simulink model "PowetrainModel"  (R2020b)
settings: Solver=VariableStepAuto  StartTime=0.0  StopTime=10.0  RelTol=1e-3
undefined symbols (not defined in the file or in its folder): sigbuilder_block
settings Model: Creator=joems  LastModifiedBy=joems

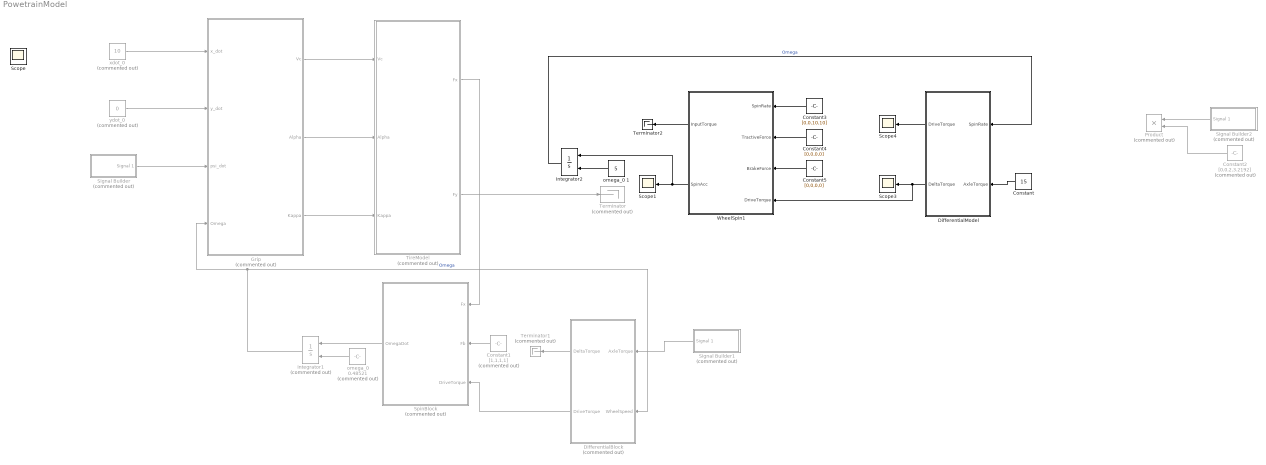
== system PowetrainModel ==
  Constant : Constant  Value=15
  Constant1 : Constant  Commented=on  Value=[1,1,1,1]
  Constant2 : Constant  Commented=on  Value=[0,0,2,3.2192]
  Constant3 : Constant  Value=[0,0,10,10]
  Constant4 : Constant  Value=[0,0,0,0]
  Constant5 : Constant  Value=[0,0,0,0]
  DifferentialBlock : MATLAB Function  Commented=on  TreatAsAtomicUnit=on
  DifferentialModel : MATLAB Function  TreatAsAtomicUnit=on
  Grip : MATLAB Function  Commented=on  TreatAsAtomicUnit=on
  Integrator1 : Integrator  Commented=on  InitialConditionSource=external
  Integrator2 : Integrator  InitialConditionSource=external
  Product : Product  Commented=on
  Scope{,1,3..4} (4 alike) : Scope
  Signal Builder : Subsystem  Tag=STV Subsys  Commented=on  LoadFcn=sigbuilder_block('load');  StartFcn=sigbuilder_block('start');  StopFcn=sigbuilder_block('stop');  ClipboardFcn=sigbuilder_block('clipboard');  mask(Sigbuilder block){tuvar=[0:10]}
      mask help: Simulink:masks:SigbuilderBlock_MD
      mask init:
      | if ~strcmp(get_param(bdroot(gcbh),'SimulationStatus'),'stopped') tuvar = sigbuilder_block('maskInit'); end
      settings: CopyFcn=sigbuilder_block('copy');  DeleteFcn=sigbuilder_block('delete');  ModelCloseFcn=sigbuilder_block('modelClose');  PreSaveFcn=sigbuilder_block('preSave');  PauseFcn=sigbuilder_block('pause');  ContinueFcn=sigbuilder_block('continue');  NameChangeFcn=sigbuilder_block('namechange');  OpenFcn=sigbuilder_block('open',[281.4 118.8 550.8 400.2 ]);  CloseFcn=sigbuilder_block('close');
      mask Display: plot(0, 0, 100, 100,[2, 2, 32, 32, 2], [68, 8, 8, 68, 68],[32, 2], [38, 38], [32, 19, 2],[53, 60, 44], [32, 17, 17, 2],[16, 16, 31, 31]);txt = getActiveGroup(gcbh);text(2, 100, txt,'verticalAlignment', 'top');
  Signal Builder1 : Subsystem  Tag=STV Subsys  Commented=on  LoadFcn=sigbuilder_block('load');  StartFcn=sigbuilder_block('start');  StopFcn=sigbuilder_block('stop');  ClipboardFcn=sigbuilder_block('clipboard');  mask(Sigbuilder block){tuvar=[0:10]}
      mask help: Simulink:masks:SigbuilderBlock_MD
      mask init:
      | if ~strcmp(get_param(bdroot(gcbh),'SimulationStatus'),'stopped') tuvar = sigbuilder_block('maskInit'); end
      settings: CopyFcn=sigbuilder_block('copy');  DeleteFcn=sigbuilder_block('delete');  ModelCloseFcn=sigbuilder_block('modelClose');  PreSaveFcn=sigbuilder_block('preSave');  PauseFcn=sigbuilder_block('pause');  ContinueFcn=sigbuilder_block('continue');  NameChangeFcn=sigbuilder_block('namechange');  OpenFcn=sigbuilder_block('open',[281.4 118.8 550.8 400.2 ]);  CloseFcn=sigbuilder_block('close');
      mask Display: plot(0, 0, 100, 100,[2, 2, 32, 32, 2], [68, 8, 8, 68, 68],[32, 2], [38, 38], [32, 19, 2],[53, 60, 44], [32, 17, 17, 2],[16, 16, 31, 31]);txt = getActiveGroup(gcbh);text(2, 100, txt,'verticalAlignment', 'top');
  Signal Builder2 : Subsystem  Tag=STV Subsys  Commented=on  LoadFcn=sigbuilder_block('load');  StartFcn=sigbuilder_block('start');  StopFcn=sigbuilder_block('stop');  ClipboardFcn=sigbuilder_block('clipboard');  mask(Sigbuilder block){tuvar=[0:10]}
      mask help: Simulink:masks:SigbuilderBlock_MD
      mask init:
      | if ~strcmp(get_param(bdroot(gcbh),'SimulationStatus'),'stopped') tuvar = sigbuilder_block('maskInit'); end
      settings: CopyFcn=sigbuilder_block('copy');  DeleteFcn=sigbuilder_block('delete');  ModelCloseFcn=sigbuilder_block('modelClose');  PreSaveFcn=sigbuilder_block('preSave');  PauseFcn=sigbuilder_block('pause');  ContinueFcn=sigbuilder_block('continue');  NameChangeFcn=sigbuilder_block('namechange');  OpenFcn=sigbuilder_block('open',[281.4 118.8 550.8 400.2 ]);  CloseFcn=sigbuilder_block('close');
      mask Display: plot(0, 0, 100, 100,[2, 2, 32, 32, 2], [68, 8, 8, 68, 68],[32, 2], [38, 38], [32, 19, 2],[53, 60, 44], [32, 17, 17, 2],[16, 16, 31, 31]);txt = getActiveGroup(gcbh);text(2, 100, txt,'verticalAlignment', 'top');
  SpinBlock : MATLAB Function  Commented=on  TreatAsAtomicUnit=on
  Terminator : Terminator  Commented=on
  Terminator1 : Terminator  Commented=on
  Terminator2 : Terminator
  TireModel : MATLAB Function  Commented=on  TreatAsAtomicUnit=on
  WheelSpin1 : MATLAB Function  TreatAsAtomicUnit=on
  "omega_0 " : Constant  Commented=on  Value=0.48521
  omega_0 1 : Constant  Value=5
  xdot_0 : Constant  Commented=on  Value=10
  ydot_0 : Constant  Commented=on  Value=0
  wires:
  Signal Builder/1(Signal 1) -> Grip/3(psi_dot)
  ydot_0/1 -> Grip/2(y_dot)
  xdot_0/1 -> Grip/1(x_dot)
  Grip/1(Vc) -> TireModel/1(Vc)
  Grip/2(Alpha) -> TireModel/2(Alpha)
  Grip/3(Kappa) -> TireModel/3(Kappa)
  TireModel/1(Fx) -> SpinBlock/1(Fx)
  SpinBlock/1(OmegaDot) -> Integrator1/1
  "omega_0 "/1 -> Integrator1/2
  Integrator1/1 -> DifferentialBlock/2(WheelSpeed), Grip/4(Omega)  "Omega"
  TireModel/2(Fy) -> Terminator/1
  Constant1/1 -> SpinBlock/2(Fb)
  Signal Builder1/1(Signal 1) -> DifferentialBlock/1(AxleTorque)
  DifferentialBlock/2(DriveTorque) -> SpinBlock/3(DriveTorque)
  DifferentialBlock/1(DeltaTorque) -> Terminator1/1
  DifferentialModel/1(DriveTorque) -> Scope4/1
  Signal Builder2/1(Signal 1) -> Product/1
  Constant2/1 -> Product/2
  Constant/1 -> DifferentialModel/2(AxleTorque)
  Constant3/1 -> WheelSpin1/1(SpinRate)
  Constant4/1 -> WheelSpin1/2(TractiveForce)
  DifferentialModel/2(DeltaTorque) -> WheelSpin1/4(DriveTorque), Scope3/1
  Constant5/1 -> WheelSpin1/3(BrakeForce)
  WheelSpin1/1(InputTorque) -> Terminator2/1
  omega_0 1/1 -> Integrator2/2
  WheelSpin1/2(SpinAcc) -> Integrator2/1, Scope1/1
  Integrator2/1 -> DifferentialModel/1(SpinRate)  "Omega"

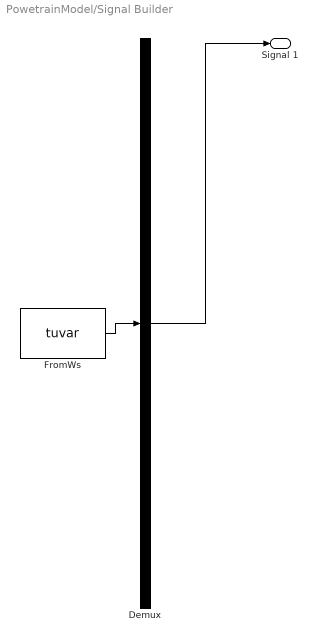
== system PowetrainModel/Signal Builder ==
  Demux : Demux  Tag=STV Demux  Outputs=1
      settings: DisplayOption=none
  FromWs : FromWorkspace  Tag=STV FromWs  VariableName=tuvar
      SigBuilderData=|
      | common.afterFinalStr = 'Extrapolate'
      | common.sampleTime = 0
      | dataSet.timeRange = [0 10]
      | dataSet.name = 'Group 1'
      | sbobj.Groups.Name = 'Group 1'
      | sbobj.Groups.Signals.Name = 'Signal 1'
      | sbobj.Groups.Signals.XData = [0 4 4.3 6 10]
      | sbobj.Groups.Signals.YData = [0 -0.005 1 1 1]
  Signal 1 : Outport  Tag=STV Outport
  wires:
  Demux/1 -> Signal 1/1
  FromWs/1 -> Demux/1

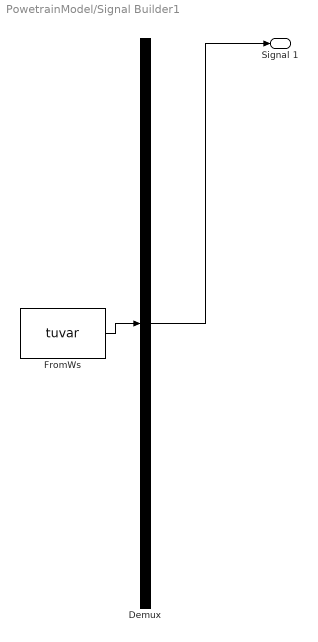
== system PowetrainModel/Signal Builder1 ==
  Demux : Demux  Tag=STV Demux  Outputs=1
      settings: DisplayOption=none
  FromWs : FromWorkspace  Tag=STV FromWs  VariableName=tuvar
      SigBuilderData=|
      | common.afterFinalStr = 'Extrapolate'
      | common.sampleTime = 0
      | dataSet.timeRange = [0 10]
      | dataSet.name = 'Group 1'
      | sbobj.Groups.Name = 'Group 1'
      | sbobj.Groups.Signals.Name = 'Signal 1'
      | sbobj.Groups.Signals.XData = [0 4 4.3 6 10]
      | sbobj.Groups.Signals.YData = [0 -0.005 1 1 1]
  Signal 1 : Outport  Tag=STV Outport
  wires:
  Demux/1 -> Signal 1/1
  FromWs/1 -> Demux/1

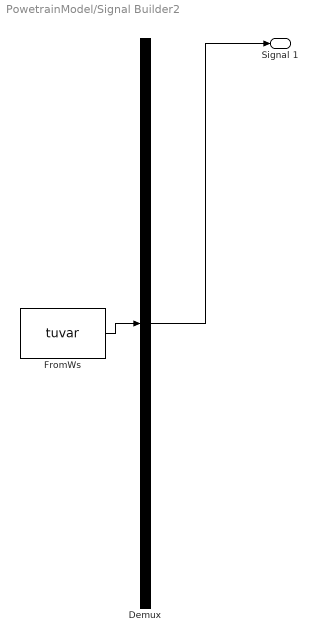
== system PowetrainModel/Signal Builder2 ==
  Demux : Demux  Tag=STV Demux  Outputs=1
      settings: DisplayOption=none
  FromWs : FromWorkspace  Tag=STV FromWs  VariableName=tuvar
      SigBuilderData=|
      | common.afterFinalStr = 'Extrapolate'
      | common.sampleTime = 0
      | dataSet.timeRange = [0 10]
      | dataSet.name = 'Group 1'
      | sbobj.Groups.Name = 'Group 1'
      | sbobj.Groups.Signals.Name = 'Signal 1'
      | sbobj.Groups.Signals.XData = [0 4 4 4.3 6 10]
      | sbobj.Groups.Signals.YData = [0 0 -0.005 1 1 1]
  Signal 1 : Outport  Tag=STV Outport
  wires:
  Demux/1 -> Signal 1/1
  FromWs/1 -> Demux/1

== matlab function PowetrainModel/TireModel ==
  data: Vc input; Alpha input; Fx output; Kappa input; Fy output
function [Fx, Fy] = TireModel(Vc, Alpha, Kappa)


Kxk = 1000;
Kya = 1000;

Fx = Kxk .* Kappa; 

Fy = Kya .* Alpha;

Vc = Vc .*1; 





 %[Fx3, Fy3,~, ~, ~] = Tire.ContactPatchLoads(Alpha, Kappa, 267/4, 12, 2, Vc, 3, Fidelity); %Check if the input values are good 

 %[Fx4, Fy4,~, ~, ~] = Tire.ContactPatchLoads(Alpha, Kappa, 267/4, 12, 2, Vc, 4, Fidelity);
 
% Fx = [Fx3, Fx4];
% Fy = [Fy3, Fy4];
end

== matlab function PowetrainModel/Grip ==
  data: x_dot input; Vc output; y_dot input; psi_dot input; Alpha output; Kappa output; Omega input; Parameter parameter
function [Vc, Alpha, Kappa]= Grip(x_dot,...
    y_dot, psi_dot, Omega, Parameter)

%% Variable Names
%x_dot0 - Intiial logetudinal velocity 
%x_dot - Logetidunal velocity
%y_dot0 - Initial lateral velocity
%y_dot Lateral velocity
%psi_dot - Yaw rate, 
%tw - Track width 
%L - Wheel Base 
%Vc3 & Vc4 - Center velocity of rear tires
%Vc3/4_x/y - Center Velocity components 


%% Center Velocity

Vc = zeros(4,2);
    % Logintidinal Center Velocity 
Vc(3,1) = x_dot - psi_dot.*(Parameter.TrackWidth/2); 

Vc(4,1) = x_dot + psi_dot.*(Parameter.TrackWidth/2);

    % Lateral Center Velocity

Vc(3,2) = y_dot - psi_dot.*Parameter.b;  

Vc(4,2) = y_dot - psi_dot.*Parameter.b;


%% Slip Angle

Alpha = zeros(1,4);

Alpha(3) = - atan2d( (y_dot - Parameter.b.*psi_dot)./ (x_dot + ...
    ( (Parameter.TrackWidth/2).*psi_dot) ), x_dot);                                            
Alpha(4) = - atan2d( (y_dot - Parameter.b.*psi_dot) ./ (x_dot - ...
    ( (Parameter.TrackWidth/2).*psi_dot) ) , x_dot);

%% Slip Ratio

Kappa = zeros(1,4); 

Kappa(3) =  (Omega*Parameter.Radius.Effective ./ Vc(3,2)*cosd(Alpha) ) - 1;

Kappa(4) = (Omega*Parameter.Radius.Effective ./ Vc(4,2)*cosd(Alpha)) - 1;


end

== matlab function PowetrainModel/SpinBlock ==
  data: Fx input; Fb input; DriveTorque input; OmegaDot output; Parameter parameter
function OmegaDot  = SpinBlock(Fx, Fb,DriveTorque, Parameter)
%% Nomenclature 
%Logentudinal Force - Fx 
%Braking Force - Fb
% Delta Torque - delT
%Torque - T
% Differential Effeciency = Nd
% Inertia of the Wheel = J 

%% Omega Acceleration

OmegaDot = zeros(1,4);

OmegaDot(3) = (Parameter.DifferentialEffeciency .*DriveTorque(3) - ...
    Fx(3).*Parameter.Radius.Effective - Fb(3).*Parameter.Radius.Rotor)...
    .* (1/Parameter.WheelInertia);

OmegaDot(4) = (Parameter.DifferentialEffeciency .*DriveTorque(4)...
    - Fx(4).*Parameter.Radius.Effective - Fb(4).*Parameter.Radius.Rotor)...
    .* (1/Parameter.WheelInertia);
end

== matlab function PowetrainModel/DifferentialBlock ==
  data: AxleTorque input; DeltaTorque output; WheelSpeed input; DriveTorque output; Parameter parameter
function [DeltaTorque, DriveTorque]= DifferentialBlock(AxleTorque, WheelSpeed,...
    Parameter)
%% Comment Header 


%% Note
%delT = (Ta/rramp) *.cot(sigma_d)).*(2/3 * ((ro^3 - ri ^3) / (ro^2
%-ro^2))(mu_c *N)*(abs(DeltaOmega)*tanh(4abs(DeltaOmega)

%% Differential Speed
DiffSpeed = WheelSpeed(3) - WheelSpeed(4);

%% Differential Torque 
DriveTorque = zeros(1,4);

if (AxleTorque > Parameter.BrakePreload) && (AxleTorque < Parameter.DrivePreload) %Is Locked 
    DeltaTorque = ( AxleTorque.*0.5).*(tanh(100*DiffSpeed)); %Insert delT here once obtained parameter values   
else 
    DeltaTorque = ( AxleTorque*0.5)*(tanh(4*DiffSpeed));   
end

DriveTorque(3) = 0.5*AxleTorque - sign(DiffSpeed)*DeltaTorque; 
DriveTorque(4) = 0.5*AxleTorque + sign(DiffSpeed)*DeltaTorque;

end

== matlab function PowetrainModel/WheelSpin1 ==
  data: InputTorque output; SpinRate input; TractiveForce input; BrakeForce input; DriveTorque input; SpinAcc output; Parameter parameter
function [InputTorque, SpinAcc]  = WheelSpin( SpinRate, ...
    TractiveForce, BrakeForce, DriveTorque, Parameter)
%% Input Bus Parsing
%SpinRate      = SpinRate; 
%TractiveForce = TractiveForce; 
%BrakeForce    = BrakeForce;
%DriveTorque   = DriveTorque;

%% Parameter Parsing
DifferentialEffec = Parameter.DifferentialEffeciency;
RotorRadius       = Parameter.Radius.Rotor;                         %Parameter.Brake.Rotor.Radius;
EffRadius         = Parameter.Radius.Effective;                     %Parameter.Tire.Radius();
Inertia           = Parameter.WheelInertia;
Damping           = Parameter.AxleDampening;
BrakeTorque       = BrakeForce .* RotorRadius;


%% Calculations
[InputTorque, SpinAcc] = WheelSpeed( SpinRate, DriveTorque, BrakeTorque, ...
    TractiveForce, EffRadius, Inertia, Damping, DifferentialEffec );

%% Output Bus Allocation	
 % SpinAcc = SpinAcc

== matlab function PowetrainModel/DifferentialModel ==
  data: SpinRate input; DriveTorque output; AxleTorque input; DeltaTorque output; Parameter parameter
function [DriveTorque, DeltaTorque] = DifferentialBlock1(SpinRate, AxleTorque, Parameter)

%% Input Bus Parsing
%SpinRate      = SpinRate; 
%TractiveForce = TractiveForce; 
%BrakeForce    = BrakeForce;
%DriveTorque   = DriveTorque;

%% Parameter Parsing
BrakePreload = Parameter.BrakePreload; %Change
DrivePreload = Parameter.DrivePreload; %Change


%% Calculations

[DriveTorque, DeltaTorque] =  DifferentialModel(SpinRate, AxleTorque, ...
    BrakePreload, DrivePreload );

%% Output Bus Allocation
%DriveTorque = DriveTorque
%DeltaTorque = DeltaTorque
